simulink model "B2B_HVDC_MMC"  (R2023b)
settings: Solver=ode23t  StartTime=0.0  StopTime=3  FixedStep=Ts_Power  MaxStep=1e-3  MinStep=Ts_Power  RelTol=1e-3
values from neighbouring files (symbols this model uses):
  AC_lim = 1*[1.5 -1.5]    [B2B_HVDC_MMC_Calc.m]
  C_pm = 10.48e-3    (= 0.01048)    [B2B_HVDC_MMC_Calc.m]
  Carm = 1.0*C_pm/n    (= 0.0002096)    [B2B_HVDC_MMC_Calc.m]    (also in HVDC_MMC_param.m = 4.88333333333e-05)
  ccsc_lim = 1*[1.0 -1.0]    [B2B_HVDC_MMC_Calc.m]
  DC_lim = 1*[1.05 -1.05]    [B2B_HVDC_MMC_Calc.m]
  f = 50    [B2B_HVDC_MMC_Calc.m]
  Fn_filter = 1000    [B2B_HVDC_MMC_Calc.m]    (also in HVDC_MMC_param.m)
  Fnom = 50    [HVDC_MMC_param.m]
  HrmOrd = N    (= 2)    [B2B_HVDC_MMC_Calc.m]    (also in HVDC_MMC_param.m)
  I_nom = S_nom/(sqrt(3)*V_grid)    [B2B_HVDC_MMC_Calc.m]
  Ireg_lim_i = 1*[1.5, -1.5]    [B2B_HVDC_MMC_Calc.m]
  Ireg_lim_r = 2*[1.5, -1.5]    [B2B_HVDC_MMC_Calc.m]
  Ki_ACreg_i = 260    [B2B_HVDC_MMC_Calc.m]
  Ki_ccsc = 5    [B2B_HVDC_MMC_Calc.m]
  Ki_DCreg_r = 150    [B2B_HVDC_MMC_Calc.m]
  Ki_Ireg_i = 200    [B2B_HVDC_MMC_Calc.m]
  Ki_Ireg_r = 50    [B2B_HVDC_MMC_Calc.m]
  Kp_ACreg_i = 2    [B2B_HVDC_MMC_Calc.m]
  Kp_ccsc = 1    [B2B_HVDC_MMC_Calc.m]
  Kp_DCreg_r = 8    [B2B_HVDC_MMC_Calc.m]
  Kp_Ireg_i = 2    [B2B_HVDC_MMC_Calc.m]
  Kp_Ireg_r = 0.8    [B2B_HVDC_MMC_Calc.m]
  L1_si = L1_pu*Z_base66/w    [B2B_HVDC_MMC_Calc.m]
  L_arm = L_arm_pu*Z_base66/w    [B2B_HVDC_MMC_Calc.m]
  L_arm_pu = 0.15    [B2B_HVDC_MMC_Calc.m]
  N = 2    [B2B_HVDC_MMC_Calc.m]
  P_nom = 220e6    (= 220000000)    [B2B_HVDC_MMC_Calc.m]
  R1_si = R1_pu*Z_base66    [B2B_HVDC_MMC_Calc.m]
  R_arm = 0.03    [B2B_HVDC_MMC_Calc.m]
  R_arm_pu = R_arm/Z_base66    [B2B_HVDC_MMC_Calc.m]
  R_load = 0.6*40    (= 24)    [B2B_HVDC_MMC_Calc.m]
  R_startup = 17    [B2B_HVDC_MMC_Calc.m]    (also in HVDC_MMC_param.m = 400)
  T_fault = 1.4    [B2B_HVDC_MMC_Calc.m]
  Ts = Ts_Power    (= 5e-05)    [B2B_HVDC_MMC_Calc.m]    (also in HVDC_MMC_param.m)
  Ts_Control = Ts_Power    (= 5e-05)    [B2B_HVDC_MMC_Calc.m]    (also in HVDC_MMC_param.m)
  Ts_DQN = MultTs*Ts_Power    (= 5e-05)    [B2B_HVDC_MMC_Calc.m]    (also in HVDC_MMC_param.m)
  Ts_Power = 1*50e-6    (= 5e-05)    [B2B_HVDC_MMC_Calc.m]    (also in HVDC_MMC_param.m)
  V_ac_ref = 1.035    [B2B_HVDC_MMC_Calc.m]
  V_grid = 66e3    (= 66000)    [B2B_HVDC_MMC_Calc.m]
  Vdc_nom = 135e3    (= 135000)    [B2B_HVDC_MMC_Calc.m]
  Vnom_prim = 333e3    (= 333000)    [HVDC_MMC_param.m]
  Xdcpnz = [zeros(6,1), Xpnz]    [B2B_HVDC_MMC_Calc.m]
  Zeta_filter = 1    [B2B_HVDC_MMC_Calc.m]    (also in HVDC_MMC_param.m)
undefined symbols (not defined in the file or in its folder): DiscIntNeverNeededParam, Pcc, Xdcpnz_c
libraries: DQN_Lib x39, simulink x26, eeTransforms x21, spsCurrentMeasurementLib x16, spsHalfBridgeMMCLib x12, spsSeriesRLCBranchLib x12, B2B_HVDC_MMC_Lib x8, spsSecondOrderFilterLib x8, spsAlphaBetaZerotodq0Lib x6, spsabctoAlphaBetaZeroLib x6, spsThreePhaseVIMeasurementLib x4, spsabctodq0Lib x3
(part 4 of 5)

== system B2B_HVDC_MMC/Dq0 Control8/Subsystem/Circulating current suppression ==
  Id_dq2- : Inport
  Enable1 : EnablePort
  Constant1 : Constant  Value=0
  Constant2 : Constant  Value=0
  Constant4 : Constant  Value=0
  Demux : Demux  Outputs=2
  Discrete PID Controller : simulink/Continuous/PID Controller  Controller=PI  Form=Parallel  TimeDomain=Discrete-time  UseExternalTs=off  SampleTime=Ts_Power  IntegratorMethod=Forward Euler  ControllerParametersSource=internal  P=Kp_ccsc  I=Ki_ccsc  D=0  UseFilter=on  N=100  TunerSelectOption=Transfer Function Based (PID Tuner App)  InitialConditionSource=internal  InitialConditionForIntegrator=0  InitialConditionForFilter=0  DifferentiatorICPrevScaledInput=0  ExternalReset=none  TrackingMode=off  Kt=1  LimitOutput=off  UpperSaturationLimit=inf  LowerSaturationLimit=-inf  LinearizeAsGain=off  AntiWindupMode=none  Kb=1  POutMin=[]  POutMax=[]  IOutMin=[]  IOutMax=[]  DOutMin=[]  DOutMax=[]  NOutMin=[]  NOutMax=[]  SumOutMin=[]  SumOutMax=[]  SaturationOutMin=[]  SaturationOutMax=[]  PParamMin=[]  PParamMax=[]  IParamMin=[]  IParamMax=[]  DParamMin=[]  DParamMax=[]  NParamMin=[]  NParamMax=[]  KbParamMin=[]  KbParamMax=[]  KtParamMin=[]  KtParamMax=[]  KbOutMin=[]  KbOutMax=[]  KtOutMin=[]  KtOutMax=[]  IntegratorOutMin=[]  IntegratorOutMax=[]  FilterOutMin=[]  FilterOutMax=[]  SumI1OutMin=[]  SumI1OutMax=[]  SumI2OutMin=[]  SumI2OutMax=[]  SumI3OutMin=[]  SumI3OutMax=[]  SumI4OutMin=[]  SumI4OutMax=[]  SumDOutMin=[]  SumDOutMax=[]  DifferentiatorOutMin=[]  DifferentiatorOutMax=[]  FilterDiffOutCoefMin=[]  FilterDiffOutCoefMax=[]  ReciprocalOutMin=[]  ReciprocalOutMax=[]  SumDenOutMin=[]  SumDenOutMax=[]  SumNumOutMin=[]  SumNumOutMax=[]  DivideOutMin=[]  DivideOutMax=[]  UdiffTsProdOutMin=[]  UdiffTsProdOutMax=[]  NTsProdOutMin=[]  NTsProdOutMax=[]  UintegralTsProdOutMin=[]  UintegralTsProdOutMax=[]  UngainTsProdOutMin=[]  UngainTsProdOutMax=[]  IntegratorContinuousStateAttributes=''  IntegratorStateMustResolveToSignalObject=off  IntegratorRTWStateStorageClass=Auto  FilterContinuousStateAttributes=''  FilterStateMustResolveToSignalObject=off  FilterRTWStateStorageClass=Auto  ParallelPVariant=InternalParameters  IdealPVariant=Disabled  IVariant=InternalParameters  DVariant=Disabled  IntegratorVariant=Discrete  SatVariant=Disabled  AWVariant=Passthrough  PCopyVariant=Disabled  TRVariant=Disabled  FdbkBlocksVariant=Forward  IdealPFdbkVariant=Disabled  SatFdbkVariant=Disabled  DerivativeFilterVariant=Disabled  NVariant=Disabled  NCopyVariant=Disabled_SignalSpec  FilterICVariant=Disabled  IntegratorICVariant=InternalICs  ExternalResetVariant=Disabled  TRSumVariant=Passthrough  SumFdbkVariant=Disabled  SumVariant=Sum_PI  TsampFilterVariant=InternalTs  TsampNgainVariant=Passthrough  TsampIntegralVariant=Passthrough
  Discrete PID Controller1 : simulink/Continuous/PID Controller  Controller=PI  Form=Parallel  TimeDomain=Discrete-time  UseExternalTs=off  SampleTime=Ts_Power  IntegratorMethod=Forward Euler  ControllerParametersSource=internal  P=Kp_ccsc  I=Ki_ccsc  D=0  UseFilter=on  N=100  TunerSelectOption=Transfer Function Based (PID Tuner App)  InitialConditionSource=internal  InitialConditionForIntegrator=0  InitialConditionForFilter=0  DifferentiatorICPrevScaledInput=0  ExternalReset=none  TrackingMode=off  Kt=1  LimitOutput=off  UpperSaturationLimit=inf  LowerSaturationLimit=-inf  LinearizeAsGain=off  AntiWindupMode=none  Kb=1  POutMin=[]  POutMax=[]  IOutMin=[]  IOutMax=[]  DOutMin=[]  DOutMax=[]  NOutMin=[]  NOutMax=[]  SumOutMin=[]  SumOutMax=[]  SaturationOutMin=[]  SaturationOutMax=[]  PParamMin=[]  PParamMax=[]  IParamMin=[]  IParamMax=[]  DParamMin=[]  DParamMax=[]  NParamMin=[]  NParamMax=[]  KbParamMin=[]  KbParamMax=[]  KtParamMin=[]  KtParamMax=[]  KbOutMin=[]  KbOutMax=[]  KtOutMin=[]  KtOutMax=[]  IntegratorOutMin=[]  IntegratorOutMax=[]  FilterOutMin=[]  FilterOutMax=[]  SumI1OutMin=[]  SumI1OutMax=[]  SumI2OutMin=[]  SumI2OutMax=[]  SumI3OutMin=[]  SumI3OutMax=[]  SumI4OutMin=[]  SumI4OutMax=[]  SumDOutMin=[]  SumDOutMax=[]  DifferentiatorOutMin=[]  DifferentiatorOutMax=[]  FilterDiffOutCoefMin=[]  FilterDiffOutCoefMax=[]  ReciprocalOutMin=[]  ReciprocalOutMax=[]  SumDenOutMin=[]  SumDenOutMax=[]  SumNumOutMin=[]  SumNumOutMax=[]  DivideOutMin=[]  DivideOutMax=[]  UdiffTsProdOutMin=[]  UdiffTsProdOutMax=[]  NTsProdOutMin=[]  NTsProdOutMax=[]  UintegralTsProdOutMin=[]  UintegralTsProdOutMax=[]  UngainTsProdOutMin=[]  UngainTsProdOutMax=[]  IntegratorContinuousStateAttributes=''  IntegratorStateMustResolveToSignalObject=off  IntegratorRTWStateStorageClass=Auto  FilterContinuousStateAttributes=''  FilterStateMustResolveToSignalObject=off  FilterRTWStateStorageClass=Auto  ParallelPVariant=InternalParameters  IdealPVariant=Disabled  IVariant=InternalParameters  DVariant=Disabled  IntegratorVariant=Discrete  SatVariant=Disabled  AWVariant=Passthrough  PCopyVariant=Disabled  TRVariant=Disabled  FdbkBlocksVariant=Forward  IdealPFdbkVariant=Disabled  SatFdbkVariant=Disabled  DerivativeFilterVariant=Disabled  NVariant=Disabled  NCopyVariant=Disabled_SignalSpec  FilterICVariant=Disabled  IntegratorICVariant=InternalICs  ExternalResetVariant=Disabled  TRSumVariant=Passthrough  SumFdbkVariant=Disabled  SumVariant=Sum_PI  TsampFilterVariant=InternalTs  TsampNgainVariant=Passthrough  TsampIntegralVariant=Passthrough
  Gain : Gain  Gain=2*L_arm_pu
  Gain1 : Gain  Gain=2*L_arm_pu
  Mux1 : Mux  Inputs=3
  Sum1 : Sum  Inputs=-+|
  Sum78 : Sum  Inputs=|++
  Sum83 : Sum  Inputs=-+|
  Sum85 : Sum  Inputs=|+-
  m_dq2 : Outport  VectorParamsAs1DForOutWhenUnconnected=off
  wires:
  Constant2/1 -> Sum85/1
  Constant4/1 -> Mux1/3
  Sum1/1 -> Mux1/2
  Discrete PID Controller1/1 -> Sum1/2
  Discrete PID Controller/1 -> Sum78/1
  Id_dq2-/1 -> Demux/1
  Gain/1 -> Sum1/1
  Sum78/1 -> Mux1/1
  Sum85/1 -> Discrete PID Controller/1
  Sum83/1 -> Discrete PID Controller1/1
  Constant1/1 -> Sum83/2
  Demux/2 -> Sum83/1, Gain1/1
  Gain1/1 -> Sum78/2
  Demux/1 -> Sum85/2, Gain/1
  Mux1/1 -> m_dq2/1

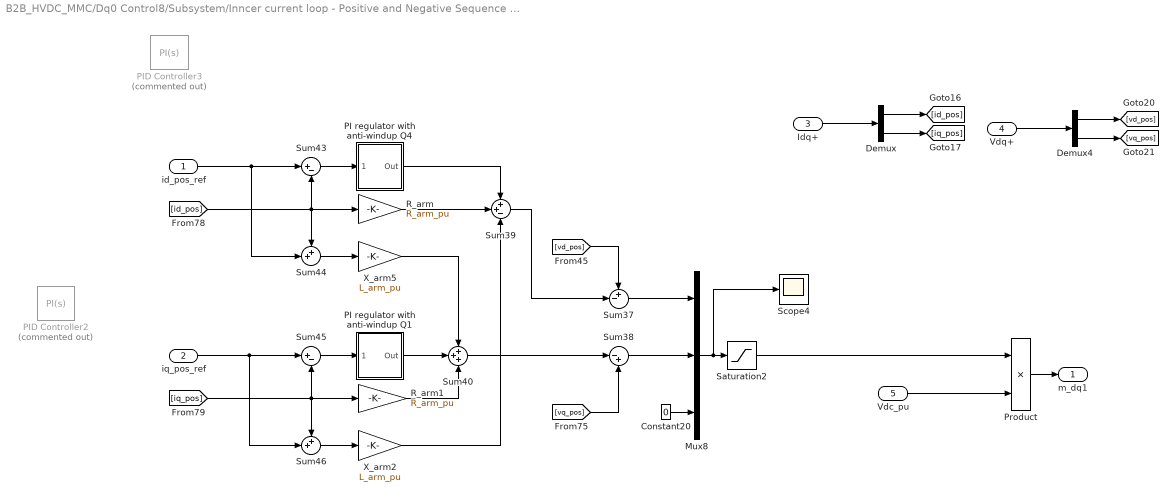
== system B2B_HVDC_MMC/Dq0 Control8/Subsystem/Inncer current loop - Positive and Negative Sequence Control ==
  id_pos_ref : Inport
  iq_pos_ref : Inport  Port=2
  Idq+ : Inport  Port=3
  Vdq+ : Inport  Port=4
  Vdc_pu : Inport  Port=5
  Constant20 : Constant  Value=0
  Demux : Demux  Outputs=2
  Demux4 : Demux  Outputs=2
  Mux8 : Mux  Inputs=3
  PI regulator with anti-windup Q1 : Subsystem  DialogController=POWERSYS.PowerSysDialog  mask(Discrete PI Controller){Kp=Kp_Ireg_i, Ki=Ki_Ireg_i, Par_Limits=[Ireg_lim_i(1) Ireg_lim_i(2)], Init=0, Ts=Ts_Control}
      mask prompts: Kp "Proportional gain (Kp):"; Ki "Integral gain (Ki):"; Par_Limits "Output limits: [ Upper   Lower ]"; Init "Output initial value:"; Ts "Sample time:"
      mask help: This block implements a discrete PI controller.
      mask init:
      | UpperLimit=Par_Limits(1);
      | LowerLimit=Par_Limits(2);
      | power_initmask();
      mask Help: This block is part of a subset of blocks in the Extras library that does not have documentation associated with it, other than the block mask description.
      mask Display: disp('PI');
  PI regulator with anti-windup Q4 : Subsystem  DialogController=POWERSYS.PowerSysDialog  mask(Discrete PI Controller){Kp=Kp_Ireg_i, Ki=Ki_Ireg_i, Par_Limits=[Ireg_lim_i(1) Ireg_lim_i(2)], Init=0, Ts=Ts_Control}
      mask prompts: Kp "Proportional gain (Kp):"; Ki "Integral gain (Ki):"; Par_Limits "Output limits: [ Upper   Lower ]"; Init "Output initial value:"; Ts "Sample time:"
      mask help: This block implements a discrete PI controller.
      mask init:
      | UpperLimit=Par_Limits(1);
      | LowerLimit=Par_Limits(2);
      | power_initmask();
      mask Help: This block is part of a subset of blocks in the Extras library that does not have documentation associated with it, other than the block mask description.
      mask Display: disp('PI');
  PID Controller2 : simulink/Continuous/PID Controller  Commented=on  Controller=PI  Form=Parallel  TimeDomain=Continuous-time  UseExternalTs=off  SampleTime=-1  IntegratorMethod=Forward Euler  ControllerParametersSource=internal  P=Kp_Ireg_i  I=Ki_Ireg_i  D=0  UseFilter=on  N=100  TunerSelectOption=Transfer Function Based (PID Tuner App)  InitialConditionSource=internal  InitialConditionForIntegrator=0  InitialConditionForFilter=0  DifferentiatorICPrevScaledInput=0  ExternalReset=none  TrackingMode=off  Kt=1  LimitOutput=off  UpperSaturationLimit=inf  LowerSaturationLimit=-inf  LinearizeAsGain=on  AntiWindupMode=none  Kb=1  POutMin=[]  POutMax=[]  IOutMin=[]  IOutMax=[]  DOutMin=[]  DOutMax=[]  NOutMin=[]  NOutMax=[]  SumOutMin=[]  SumOutMax=[]  SaturationOutMin=[]  SaturationOutMax=[]  PParamMin=[]  PParamMax=[]  IParamMin=[]  IParamMax=[]  DParamMin=[]  DParamMax=[]  NParamMin=[]  NParamMax=[]  KbParamMin=[]  KbParamMax=[]  KtParamMin=[]  KtParamMax=[]  KbOutMin=[]  KbOutMax=[]  KtOutMin=[]  KtOutMax=[]  IntegratorOutMin=[]  IntegratorOutMax=[]  FilterOutMin=[]  FilterOutMax=[]  SumI1OutMin=[]  SumI1OutMax=[]  SumI2OutMin=[]  SumI2OutMax=[]  SumI3OutMin=[]  SumI3OutMax=[]  SumI4OutMin=[]  SumI4OutMax=[]  SumDOutMin=[]  SumDOutMax=[]  DifferentiatorOutMin=[]  DifferentiatorOutMax=[]  FilterDiffOutCoefMin=[]  FilterDiffOutCoefMax=[]  ReciprocalOutMin=[]  ReciprocalOutMax=[]  SumDenOutMin=[]  SumDenOutMax=[]  SumNumOutMin=[]  SumNumOutMax=[]  DivideOutMin=[]  DivideOutMax=[]  UdiffTsProdOutMin=[]  UdiffTsProdOutMax=[]  NTsProdOutMin=[]  NTsProdOutMax=[]  UintegralTsProdOutMin=[]  UintegralTsProdOutMax=[]  UngainTsProdOutMin=[]  UngainTsProdOutMax=[]  IntegratorContinuousStateAttributes=''  IntegratorStateMustResolveToSignalObject=off  IntegratorRTWStateStorageClass=Auto  FilterContinuousStateAttributes=''  FilterStateMustResolveToSignalObject=off  FilterRTWStateStorageClass=Auto  ParallelPVariant=InternalParameters  IdealPVariant=Disabled  IVariant=InternalParameters  DVariant=Disabled  IntegratorVariant=Continuous  SatVariant=Disabled  AWVariant=Passthrough  PCopyVariant=Disabled  TRVariant=Disabled  FdbkBlocksVariant=Forward  IdealPFdbkVariant=Disabled  SatFdbkVariant=Disabled  DerivativeFilterVariant=Disabled  NVariant=Disabled  NCopyVariant=Disabled_SignalSpec  FilterICVariant=Disabled  IntegratorICVariant=InternalICs  ExternalResetVariant=Disabled  TRSumVariant=Passthrough  SumFdbkVariant=Disabled  SumVariant=Sum_PI  TsampFilterVariant=InternalTs  TsampNgainVariant=Passthrough  TsampIntegralVariant=Passthrough
  PID Controller3 : simulink/Continuous/PID Controller  Commented=on  Controller=PI  Form=Parallel  TimeDomain=Continuous-time  UseExternalTs=off  SampleTime=-1  IntegratorMethod=Forward Euler  ControllerParametersSource=internal  P=Kp_Ireg_i  I=Ki_Ireg_i  D=0  UseFilter=on  N=100  TunerSelectOption=Transfer Function Based (PID Tuner App)  InitialConditionSource=internal  InitialConditionForIntegrator=0  InitialConditionForFilter=0  DifferentiatorICPrevScaledInput=0  ExternalReset=none  TrackingMode=off  Kt=1  LimitOutput=off  UpperSaturationLimit=inf  LowerSaturationLimit=-inf  LinearizeAsGain=on  AntiWindupMode=none  Kb=1  POutMin=[]  POutMax=[]  IOutMin=[]  IOutMax=[]  DOutMin=[]  DOutMax=[]  NOutMin=[]  NOutMax=[]  SumOutMin=[]  SumOutMax=[]  SaturationOutMin=[]  SaturationOutMax=[]  PParamMin=[]  PParamMax=[]  IParamMin=[]  IParamMax=[]  DParamMin=[]  DParamMax=[]  NParamMin=[]  NParamMax=[]  KbParamMin=[]  KbParamMax=[]  KtParamMin=[]  KtParamMax=[]  KbOutMin=[]  KbOutMax=[]  KtOutMin=[]  KtOutMax=[]  IntegratorOutMin=[]  IntegratorOutMax=[]  FilterOutMin=[]  FilterOutMax=[]  SumI1OutMin=[]  SumI1OutMax=[]  SumI2OutMin=[]  SumI2OutMax=[]  SumI3OutMin=[]  SumI3OutMax=[]  SumI4OutMin=[]  SumI4OutMax=[]  SumDOutMin=[]  SumDOutMax=[]  DifferentiatorOutMin=[]  DifferentiatorOutMax=[]  FilterDiffOutCoefMin=[]  FilterDiffOutCoefMax=[]  ReciprocalOutMin=[]  ReciprocalOutMax=[]  SumDenOutMin=[]  SumDenOutMax=[]  SumNumOutMin=[]  SumNumOutMax=[]  DivideOutMin=[]  DivideOutMax=[]  UdiffTsProdOutMin=[]  UdiffTsProdOutMax=[]  NTsProdOutMin=[]  NTsProdOutMax=[]  UintegralTsProdOutMin=[]  UintegralTsProdOutMax=[]  UngainTsProdOutMin=[]  UngainTsProdOutMax=[]  IntegratorContinuousStateAttributes=''  IntegratorStateMustResolveToSignalObject=off  IntegratorRTWStateStorageClass=Auto  FilterContinuousStateAttributes=''  FilterStateMustResolveToSignalObject=off  FilterRTWStateStorageClass=Auto  ParallelPVariant=InternalParameters  IdealPVariant=Disabled  IVariant=InternalParameters  DVariant=Disabled  IntegratorVariant=Continuous  SatVariant=Disabled  AWVariant=Passthrough  PCopyVariant=Disabled  TRVariant=Disabled  FdbkBlocksVariant=Forward  IdealPFdbkVariant=Disabled  SatFdbkVariant=Disabled  DerivativeFilterVariant=Disabled  NVariant=Disabled  NCopyVariant=Disabled_SignalSpec  FilterICVariant=Disabled  IntegratorICVariant=InternalICs  ExternalResetVariant=Disabled  TRSumVariant=Passthrough  SumFdbkVariant=Disabled  SumVariant=Sum_PI  TsampFilterVariant=InternalTs  TsampNgainVariant=Passthrough  TsampIntegralVariant=Passthrough
  Product : Product
  R_arm : Gain  Gain=R_arm_pu
  R_arm1 : Gain  Gain=R_arm_pu
  Saturation2 : Saturate  UpperLimit=Ireg_lim_i(1)  LowerLimit=Ireg_lim_i(2)
  Scope4 : Scope
  Sum37 : Sum  Inputs=+-|
  Sum38 : Sum  Inputs=|-+
  Sum39 : Sum  Inputs=++-
  Sum40 : Sum  Inputs=+++
  Sum43 : Sum  Inputs=|+-
  Sum44 : Sum  Inputs=++|
  Sum45 : Sum  Inputs=|+-
  Sum46 : Sum  Inputs=++|
  X_arm2 : Gain  Gain=L_arm_pu
  X_arm5 : Gain  Gain=L_arm_pu
  m_dq1 : Outport  VectorParamsAs1DForOutWhenUnconnected=off
  wires:
  Mux8/1 -> Scope4/1, Saturation2/1
  Vdq+/1 -> Demux4/1
  Idq+/1 -> Demux/1
  [id_pos] -> Sum44/1, Sum43/2, R_arm/1
  Demux4/2 -> [vq_pos]
  Demux4/1 -> [vd_pos]
  Demux/1 -> [id_pos]
  Demux/2 -> [iq_pos]
  Sum45/1 -> PI regulator with anti-windup Q1/1(Error)
  Sum37/1 -> Mux8/1
  iq_pos_ref/1 -> Sum45/1, Sum46/2
  Sum40/1 -> Sum38/1
  X_arm2/1 -> Sum39/3
  R_arm1/1 -> Sum40/3
  R_arm/1 -> Sum39/2
  Sum44/1 -> X_arm5/1
  Sum43/1 -> PI regulator with anti-windup Q4/1(Error)
  Sum46/1 -> X_arm2/1
  Sum38/1 -> Mux8/2
  [vd_pos] -> Sum37/1
  [vq_pos] -> Sum38/2
  X_arm5/1 -> Sum40/1
  Sum39/1 -> Sum37/2
  id_pos_ref/1 -> Sum43/1, Sum44/2
  PI regulator with anti-windup Q1/1(Out) -> Sum40/2
  Constant20/1 -> Mux8/3
  [iq_pos] -> Sum45/2, Sum46/1, R_arm1/1
  PI regulator with anti-windup Q4/1(Out) -> Sum39/1
  Vdc_pu/1 -> Product/2
  Saturation2/1 -> Product/1
  Product/1 -> m_dq1/1

== system B2B_HVDC_MMC/Dq0 Control8/Subsystem/Outer loop - AC RMS controller1 ==
  Vac_ref : Inport
  vdq+ : Inport  Port=2
  Enable : Inport  Port=3
  PI regulator with anti-windup Q1 : Subsystem  DialogController=POWERSYS.PowerSysDialog  mask(Discrete PI Controller){Kp=Kp_ACreg_i, Ki=Ki_ACreg_i, Par_Limits=[AC_lim(1) AC_lim(2)], Init=0, Ts=Ts_Control}
      mask prompts: Kp "Proportional gain (Kp):"; Ki "Integral gain (Ki):"; Par_Limits "Output limits: [ Upper   Lower ]"; Init "Output initial value:"; Ts "Sample time:"
      mask help: This block implements a discrete PI controller.
      mask init:
      | UpperLimit=Par_Limits(1);
      | LowerLimit=Par_Limits(2);
      | power_initmask();
      mask Help: This block is part of a subset of blocks in the Extras library that does not have documentation associated with it, other than the block mask description.
      mask Display: disp('PI');
  Selector : Selector  InputPortWidth=2  IndexOptions=Index vector (dialog)  Indices=[1]  OutputSizes=1
  Sum1 : Sum  Inputs=|+-
  Switch1 : Switch  Criteria=u2 > Threshold  Threshold=0.5  OutDataTypeStr=double  SaturateOnIntegerOverflow=off  InputSameDT=off
  Id_ref : Outport  VectorParamsAs1DForOutWhenUnconnected=off
  wires:
  vdq+/1 -> Selector/1
  Sum1/1 -> PI regulator with anti-windup Q1/1(Error)
  Enable/1 -> Switch1/2
  Switch1/1 -> Sum1/1
  Vac_ref/1 -> Switch1/1
  PI regulator with anti-windup Q1/1(Out) -> [Idp_ref], Id_ref/1
  Selector/1 -> Switch1/3, Sum1/2

== system B2B_HVDC_MMC/Dq0 Control8/Subsystem/Reactive power Set-point ==
  T_Qreg_on : Inport
  Q_ref : Inport  Port=2
  Vdq+ : Inport  Port=3
  Enable : EnablePort
  Constant : Constant  Value=0
  Constant1 : Constant
  Constant2 : Constant  Value=0.75
  Divide : Product  Inputs=*/
  Gain3 : Gain  Gain=-1
  Rate Transition9 : RateTransition  Commented=on  OutPortSampleTime=Ts_Control
  Scope : Scope  NumInputPorts=4
  Selector : Selector  InputPortWidth=2  IndexOptions=Index vector (dialog)  Indices=[1]  OutputSizes=1
  Selector1 : Selector  InputPortWidth=2  IndexOptions=Index vector (dialog)  Indices=[2]  OutputSizes=1
  Switch : Switch  Criteria=u2 > Threshold  SaturateOnIntegerOverflow=off  InputSameDT=off
  Switch1 : Switch  Criteria=u2 > Threshold  SaturateOnIntegerOverflow=off  InputSameDT=off
  Switch2 : Switch  Criteria=u2 > Threshold  Threshold=0.65  SaturateOnIntegerOverflow=off  InputSameDT=off
  Unit Delay6 : UnitDelay  Commented=on  SampleTime=Ts_Power  HasFrameUpgradeWarning=on
  Iq_ref : Outport  VectorParamsAs1DForOutWhenUnconnected=off
  wires:
  Switch/1 -> Divide/1
  Vdq+/1 -> Selector/1
  Switch1/1 -> Divide/2, Scope/2
  Constant/1 -> Switch/3
  Divide/1 -> Gain3/1
  Selector1/1 -> Switch/1
  Q_ref/1 -> Selector1/1
  Constant1/1 -> Switch1/3
  T_Qreg_on/1 -> Switch1/2, Switch/2
  Constant2/1 -> Switch2/3
  Selector/1 -> Switch2/2, Switch2/1, Scope/3
  Unit Delay6/1 -> Rate Transition9/1
  Gain3/1 -> Scope/1, [Iqp_ref], Iq_ref/1
  Switch2/1 -> Switch1/1

== system B2B_HVDC_MMC/Dq0 Control11/Subsystem1/DC voltage control - Outer loop/PI regulator with anti-windup Q ==
  note: Anti-windup mechanism: Method of conditionnal integration
      |
      | The integration is suspended if saturation occurs and the
      | control error is of the same sign as the control signal.
      |
      | [1] L.Rundqwist, "Anti-Reset Windup for PID Controllers," Ph.D. Thesis TRFT-1033,
      | Departement of Automatic Control, Lund Institute of Technology, Lund, Sweeden, 1991.
  note: Modified by Tony - Adding controllable saturation operation for fault handling.
  Error : Inport  SampleTime=Ts
  Limit : Inport  Port=2
  Compare To Zero : simulink/Logic and Bit Operations/Compare To Zero  relop=>  OutDataTypeStr=uint8  ZeroCross=off
  Compare To Zero1 : simulink/Logic and Bit Operations/Compare To Zero  relop=<  OutDataTypeStr=uint8  ZeroCross=off
  Constant : Constant  Value=0
  Constant2 : Constant  Value=UpperLimit
  Constant3 : Constant  Value=LowerLimit
  Demux : Demux  Outputs=2
  Discrete-Time Integrator1 : DiscreteIntegrator  IntegratorMethod=Integration: Trapezoidal  InitialCondition=Init  SampleTime=Ts  LimitOutput=on  UpperSaturationLimit=UpperLimit  LowerSaturationLimit=LowerLimit  ShowStatePort=on  ICPrevOutput=DiscIntNeverNeededParam  ICPrevScaledInput=DiscIntNeverNeededParam
  Kp4 : Gain  Gain=Kp  SaturateOnIntegerOverflow=on  SampleTime=Ts  OutDataTypeStr=Inherit: Same as input  ParamDataTypeStr=Inherit: Same as input
  Kp5 : Gain  Gain=Ki  SaturateOnIntegerOverflow=on  SampleTime=Ts  OutDataTypeStr=Inherit: Same as input  ParamDataTypeStr=Inherit: Same as input
  Logical Operator : Logic  AllPortsSameDT=off  OutDataTypeStr=boolean
  Logical Operator1 : Logic  AllPortsSameDT=off  OutDataTypeStr=boolean
  Logical Operator2 : Logic  Operator=OR  AllPortsSameDT=off  OutDataTypeStr=boolean
  Relational Operator : RelationalOperator  OutDataTypeStr=boolean  InputSameDT=off
  Relational Operator1 : RelationalOperator  Operator=<=  OutDataTypeStr=boolean  InputSameDT=off
  Saturation Dynamic1 : simulink/Discontinuities/Saturation Dynamic  OutMin=[]  OutMax=[]  OutDataTypeStr=Inherit: Same as second input  OutDataType=fixdt(1, 16)  OutScaling=2^-10  DoSatur=off
  Sum1 : Sum  InputSameDT=on  SaturateOnIntegerOverflow=on  SampleTime=Ts  OutDataTypeStr=Inherit: Same as first input
  Sum6 : Sum  InputSameDT=on  SaturateOnIntegerOverflow=on  SampleTime=Ts  OutDataTypeStr=Inherit: Same as first input
  Switch : Switch  Criteria=u2 > Threshold  SaturateOnIntegerOverflow=off  InputSameDT=off
  Zero-Order Hold : ZeroOrderHold  SampleTime=Ts
  Out : Outport  SampleTime=Ts  InitialOutput=0  VectorParamsAs1DForOutWhenUnconnected=off
  wires:
  Constant3/1 -> Relational Operator1/2
  Constant2/1 -> Relational Operator/2
  Saturation Dynamic1/1 -> Out/1
  Sum6/1 -> Saturation Dynamic1/2
  Discrete-Time Integrator1/State -> Sum1/1
  Discrete-Time Integrator1/1 -> Sum6/2
  Constant/1 -> Switch/1
  Zero-Order Hold/1 -> Sum1/2, Sum6/1
  Sum1/1 -> Relational Operator1/1, Relational Operator/1
  Logical Operator2/1 -> Switch/2
  Relational Operator/1 -> Logical Operator/1  "UpperLimit_is_Reached"
  Relational Operator1/1 -> Logical Operator1/1  "LowerLimit_Is_Reached"
  Compare To Zero/1 -> Logical Operator/2  "Error_is_positive"
  Logical Operator/1 -> Logical Operator2/1
  Logical Operator1/1 -> Logical Operator2/2
  Compare To Zero1/1 -> Logical Operator1/2  "Error_is_negative"
  Error/1 -> Compare To Zero1/1, Compare To Zero/1, Kp4/1, Kp5/1
  Kp4/1 -> Zero-Order Hold/1
  Switch/1 -> Discrete-Time Integrator1/1
  Kp5/1 -> Switch/3
  Limit/1 -> Demux/1
  Demux/1 -> Saturation Dynamic1/1
  Demux/2 -> Saturation Dynamic1/3

== system B2B_HVDC_MMC/Dq0 Control11/Subsystem1/Inncer current loop - Positive and Negative Sequence Control/PI regulator with anti-windup Q1 ==
  note: Anti-windup mechanism: Method of conditionnal integration
      |
      | The integration is suspended if saturation occurs and the
      | control error is of the same sign as the control signal.
      |
      | [1] L.Rundqwist, "Anti-Reset Windup for PID Controllers," Ph.D. Thesis TRFT-1033,
      | Departement of Automatic Control, Lund Institute of Technology, Lund, Sweeden, 1991.
  Error : Inport  SampleTime=Ts
  Compare To Zero : simulink/Logic and Bit Operations/Compare To Zero  relop=>  OutDataTypeStr=uint8  ZeroCross=off
  Compare To Zero1 : simulink/Logic and Bit Operations/Compare To Zero  relop=<  OutDataTypeStr=uint8  ZeroCross=off
  Constant : Constant  Value=0
  Constant1 : Constant  Value=UpperLimit
  Constant3 : Constant  Value=LowerLimit
  Discrete-Time Integrator : DiscreteIntegrator  IntegratorMethod=Integration: Trapezoidal  InitialCondition=Init  SampleTime=Ts  LimitOutput=on  UpperSaturationLimit=UpperLimit  LowerSaturationLimit=LowerLimit  ShowStatePort=on  ICPrevOutput=DiscIntNeverNeededParam  ICPrevScaledInput=DiscIntNeverNeededParam
  Kp4 : Gain  Gain=Kp  SaturateOnIntegerOverflow=on  SampleTime=Ts  OutDataTypeStr=Inherit: Same as input  ParamDataTypeStr=Inherit: Same as input
  Kp5 : Gain  Gain=Ki  SaturateOnIntegerOverflow=on  SampleTime=Ts  OutDataTypeStr=Inherit: Same as input  ParamDataTypeStr=Inherit: Same as input
  Logical Operator : Logic  AllPortsSameDT=off  OutDataTypeStr=boolean
  Logical Operator1 : Logic  AllPortsSameDT=off  OutDataTypeStr=boolean
  Logical Operator2 : Logic  Operator=OR  AllPortsSameDT=off  OutDataTypeStr=boolean
  Relational Operator : RelationalOperator  OutDataTypeStr=boolean  InputSameDT=off
  Relational Operator1 : RelationalOperator  Operator=<=  OutDataTypeStr=boolean  InputSameDT=off
  Saturation2 : Saturate  UpperLimit=UpperLimit  LowerLimit=LowerLimit  SampleTime=Ts
  Sum1 : Sum  InputSameDT=on  SaturateOnIntegerOverflow=on  SampleTime=Ts  OutDataTypeStr=Inherit: Same as first input
  Sum6 : Sum  InputSameDT=on  SaturateOnIntegerOverflow=on  SampleTime=Ts  OutDataTypeStr=Inherit: Same as first input
  Switch : Switch  Criteria=u2 > Threshold  SaturateOnIntegerOverflow=off  InputSameDT=off
  Zero-Order Hold : ZeroOrderHold  SampleTime=Ts
  Out : Outport  SampleTime=Ts  InitialOutput=0  VectorParamsAs1DForOutWhenUnconnected=off
  wires:
  Kp5/1 -> Switch/3
  Switch/1 -> Discrete-Time Integrator/1
  Saturation2/1 -> Out/1
  Discrete-Time Integrator/1 -> Sum6/2
  Kp4/1 -> Zero-Order Hold/1
  Sum6/1 -> Saturation2/1
  Error/1 -> Kp5/1, Kp4/1, Compare To Zero/1, Compare To Zero1/1
  Compare To Zero1/1 -> Logical Operator1/2  "Error_is_negative"
  Logical Operator1/1 -> Logical Operator2/2
  Logical Operator/1 -> Logical Operator2/1
  Compare To Zero/1 -> Logical Operator/2  "Error_is_positive"
  Constant3/1 -> Relational Operator1/2
  Constant1/1 -> Relational Operator/2
  Relational Operator1/1 -> Logical Operator1/1  "LowerLimit_Is_Reached"
  Relational Operator/1 -> Logical Operator/1  "UpperLimit_is_Reached"
  Logical Operator2/1 -> Switch/2
  Sum1/1 -> Relational Operator/1, Relational Operator1/1
  Discrete-Time Integrator/State -> Sum1/1
  Zero-Order Hold/1 -> Sum6/1, Sum1/2
  Constant/1 -> Switch/1

== system B2B_HVDC_MMC/Dq0 Control11/Subsystem1/Inncer current loop - Positive and Negative Sequence Control/PI regulator with anti-windup Q4 ==
  note: Anti-windup mechanism: Method of conditionnal integration
      |
      | The integration is suspended if saturation occurs and the
      | control error is of the same sign as the control signal.
      |
      | [1] L.Rundqwist, "Anti-Reset Windup for PID Controllers," Ph.D. Thesis TRFT-1033,
      | Departement of Automatic Control, Lund Institute of Technology, Lund, Sweeden, 1991.
  Error : Inport  SampleTime=Ts
  Compare To Zero : simulink/Logic and Bit Operations/Compare To Zero  relop=>  OutDataTypeStr=uint8  ZeroCross=off
  Compare To Zero1 : simulink/Logic and Bit Operations/Compare To Zero  relop=<  OutDataTypeStr=uint8  ZeroCross=off
  Constant : Constant  Value=0
  Constant1 : Constant  Value=UpperLimit
  Constant3 : Constant  Value=LowerLimit
  Discrete-Time Integrator : DiscreteIntegrator  IntegratorMethod=Integration: Trapezoidal  InitialCondition=Init  SampleTime=Ts  LimitOutput=on  UpperSaturationLimit=UpperLimit  LowerSaturationLimit=LowerLimit  ShowStatePort=on  ICPrevOutput=DiscIntNeverNeededParam  ICPrevScaledInput=DiscIntNeverNeededParam
  Kp4 : Gain  Gain=Kp  SaturateOnIntegerOverflow=on  SampleTime=Ts  OutDataTypeStr=Inherit: Same as input  ParamDataTypeStr=Inherit: Same as input
  Kp5 : Gain  Gain=Ki  SaturateOnIntegerOverflow=on  SampleTime=Ts  OutDataTypeStr=Inherit: Same as input  ParamDataTypeStr=Inherit: Same as input
  Logical Operator : Logic  AllPortsSameDT=off  OutDataTypeStr=boolean
  Logical Operator1 : Logic  AllPortsSameDT=off  OutDataTypeStr=boolean
  Logical Operator2 : Logic  Operator=OR  AllPortsSameDT=off  OutDataTypeStr=boolean
  Relational Operator : RelationalOperator  OutDataTypeStr=boolean  InputSameDT=off
  Relational Operator1 : RelationalOperator  Operator=<=  OutDataTypeStr=boolean  InputSameDT=off
  Saturation2 : Saturate  UpperLimit=UpperLimit  LowerLimit=LowerLimit  SampleTime=Ts
  Sum1 : Sum  InputSameDT=on  SaturateOnIntegerOverflow=on  SampleTime=Ts  OutDataTypeStr=Inherit: Same as first input
  Sum6 : Sum  InputSameDT=on  SaturateOnIntegerOverflow=on  SampleTime=Ts  OutDataTypeStr=Inherit: Same as first input
  Switch : Switch  Criteria=u2 > Threshold  SaturateOnIntegerOverflow=off  InputSameDT=off
  Zero-Order Hold : ZeroOrderHold  SampleTime=Ts
  Out : Outport  SampleTime=Ts  InitialOutput=0  VectorParamsAs1DForOutWhenUnconnected=off
  wires:
  Kp5/1 -> Switch/3
  Switch/1 -> Discrete-Time Integrator/1
  Saturation2/1 -> Out/1
  Discrete-Time Integrator/1 -> Sum6/2
  Kp4/1 -> Zero-Order Hold/1
  Sum6/1 -> Saturation2/1
  Error/1 -> Kp5/1, Kp4/1, Compare To Zero/1, Compare To Zero1/1
  Compare To Zero1/1 -> Logical Operator1/2  "Error_is_negative"
  Logical Operator1/1 -> Logical Operator2/2
  Logical Operator/1 -> Logical Operator2/1
  Compare To Zero/1 -> Logical Operator/2  "Error_is_positive"
  Constant3/1 -> Relational Operator1/2
  Constant1/1 -> Relational Operator/2
  Relational Operator1/1 -> Logical Operator1/1  "LowerLimit_Is_Reached"
  Relational Operator/1 -> Logical Operator/1  "UpperLimit_is_Reached"
  Logical Operator2/1 -> Switch/2
  Sum1/1 -> Relational Operator/1, Relational Operator1/1
  Discrete-Time Integrator/State -> Sum1/1
  Zero-Order Hold/1 -> Sum6/1, Sum1/2
  Constant/1 -> Switch/1

== system B2B_HVDC_MMC/Dq0 Control8/Subsystem/Inncer current loop - Positive and Negative Sequence Control/PI regulator with anti-windup Q1 ==
  note: Anti-windup mechanism: Method of conditionnal integration
      |
      | The integration is suspended if saturation occurs and the
      | control error is of the same sign as the control signal.
      |
      | [1] L.Rundqwist, "Anti-Reset Windup for PID Controllers," Ph.D. Thesis TRFT-1033,
      | Departement of Automatic Control, Lund Institute of Technology, Lund, Sweeden, 1991.
  Error : Inport  SampleTime=Ts
  Compare To Zero : simulink/Logic and Bit Operations/Compare To Zero  relop=>  OutDataTypeStr=uint8  ZeroCross=off
  Compare To Zero1 : simulink/Logic and Bit Operations/Compare To Zero  relop=<  OutDataTypeStr=uint8  ZeroCross=off
  Constant : Constant  Value=0
  Constant1 : Constant  Value=UpperLimit
  Constant3 : Constant  Value=LowerLimit
  Discrete-Time Integrator : DiscreteIntegrator  IntegratorMethod=Integration: Trapezoidal  InitialCondition=Init  SampleTime=Ts  LimitOutput=on  UpperSaturationLimit=UpperLimit  LowerSaturationLimit=LowerLimit  ShowStatePort=on  ICPrevOutput=DiscIntNeverNeededParam  ICPrevScaledInput=DiscIntNeverNeededParam
  Kp4 : Gain  Gain=Kp  SaturateOnIntegerOverflow=on  SampleTime=Ts  OutDataTypeStr=Inherit: Same as input  ParamDataTypeStr=Inherit: Same as input
  Kp5 : Gain  Gain=Ki  SaturateOnIntegerOverflow=on  SampleTime=Ts  OutDataTypeStr=Inherit: Same as input  ParamDataTypeStr=Inherit: Same as input
  Logical Operator : Logic  AllPortsSameDT=off  OutDataTypeStr=boolean
  Logical Operator1 : Logic  AllPortsSameDT=off  OutDataTypeStr=boolean
  Logical Operator2 : Logic  Operator=OR  AllPortsSameDT=off  OutDataTypeStr=boolean
  Relational Operator : RelationalOperator  OutDataTypeStr=boolean  InputSameDT=off
  Relational Operator1 : RelationalOperator  Operator=<=  OutDataTypeStr=boolean  InputSameDT=off
  Saturation2 : Saturate  UpperLimit=UpperLimit  LowerLimit=LowerLimit  SampleTime=Ts
  Sum1 : Sum  InputSameDT=on  SaturateOnIntegerOverflow=on  SampleTime=Ts  OutDataTypeStr=Inherit: Same as first input
  Sum6 : Sum  InputSameDT=on  SaturateOnIntegerOverflow=on  SampleTime=Ts  OutDataTypeStr=Inherit: Same as first input
  Switch : Switch  Criteria=u2 > Threshold  SaturateOnIntegerOverflow=off  InputSameDT=off
  Zero-Order Hold : ZeroOrderHold  SampleTime=Ts
  Out : Outport  SampleTime=Ts  InitialOutput=0  VectorParamsAs1DForOutWhenUnconnected=off
  wires:
  Kp5/1 -> Switch/3
  Switch/1 -> Discrete-Time Integrator/1
  Saturation2/1 -> Out/1
  Discrete-Time Integrator/1 -> Sum6/2
  Kp4/1 -> Zero-Order Hold/1
  Sum6/1 -> Saturation2/1
  Error/1 -> Kp5/1, Kp4/1, Compare To Zero/1, Compare To Zero1/1
  Compare To Zero1/1 -> Logical Operator1/2  "Error_is_negative"
  Logical Operator1/1 -> Logical Operator2/2
  Logical Operator/1 -> Logical Operator2/1
  Compare To Zero/1 -> Logical Operator/2  "Error_is_positive"
  Constant3/1 -> Relational Operator1/2
  Constant1/1 -> Relational Operator/2
  Relational Operator1/1 -> Logical Operator1/1  "LowerLimit_Is_Reached"
  Relational Operator/1 -> Logical Operator/1  "UpperLimit_is_Reached"
  Logical Operator2/1 -> Switch/2
  Sum1/1 -> Relational Operator/1, Relational Operator1/1
  Discrete-Time Integrator/State -> Sum1/1
  Zero-Order Hold/1 -> Sum6/1, Sum1/2
  Constant/1 -> Switch/1

== system B2B_HVDC_MMC/Dq0 Control8/Subsystem/Inncer current loop - Positive and Negative Sequence Control/PI regulator with anti-windup Q4 ==
  note: Anti-windup mechanism: Method of conditionnal integration
      |
      | The integration is suspended if saturation occurs and the
      | control error is of the same sign as the control signal.
      |
      | [1] L.Rundqwist, "Anti-Reset Windup for PID Controllers," Ph.D. Thesis TRFT-1033,
      | Departement of Automatic Control, Lund Institute of Technology, Lund, Sweeden, 1991.
  Error : Inport  SampleTime=Ts
  Compare To Zero : simulink/Logic and Bit Operations/Compare To Zero  relop=>  OutDataTypeStr=uint8  ZeroCross=off
  Compare To Zero1 : simulink/Logic and Bit Operations/Compare To Zero  relop=<  OutDataTypeStr=uint8  ZeroCross=off
  Constant : Constant  Value=0
  Constant1 : Constant  Value=UpperLimit
  Constant3 : Constant  Value=LowerLimit
  Discrete-Time Integrator : DiscreteIntegrator  IntegratorMethod=Integration: Trapezoidal  InitialCondition=Init  SampleTime=Ts  LimitOutput=on  UpperSaturationLimit=UpperLimit  LowerSaturationLimit=LowerLimit  ShowStatePort=on  ICPrevOutput=DiscIntNeverNeededParam  ICPrevScaledInput=DiscIntNeverNeededParam
  Kp4 : Gain  Gain=Kp  SaturateOnIntegerOverflow=on  SampleTime=Ts  OutDataTypeStr=Inherit: Same as input  ParamDataTypeStr=Inherit: Same as input
  Kp5 : Gain  Gain=Ki  SaturateOnIntegerOverflow=on  SampleTime=Ts  OutDataTypeStr=Inherit: Same as input  ParamDataTypeStr=Inherit: Same as input
  Logical Operator : Logic  AllPortsSameDT=off  OutDataTypeStr=boolean
  Logical Operator1 : Logic  AllPortsSameDT=off  OutDataTypeStr=boolean
  Logical Operator2 : Logic  Operator=OR  AllPortsSameDT=off  OutDataTypeStr=boolean
  Relational Operator : RelationalOperator  OutDataTypeStr=boolean  InputSameDT=off
  Relational Operator1 : RelationalOperator  Operator=<=  OutDataTypeStr=boolean  InputSameDT=off
  Saturation2 : Saturate  UpperLimit=UpperLimit  LowerLimit=LowerLimit  SampleTime=Ts
  Sum1 : Sum  InputSameDT=on  SaturateOnIntegerOverflow=on  SampleTime=Ts  OutDataTypeStr=Inherit: Same as first input
  Sum6 : Sum  InputSameDT=on  SaturateOnIntegerOverflow=on  SampleTime=Ts  OutDataTypeStr=Inherit: Same as first input
  Switch : Switch  Criteria=u2 > Threshold  SaturateOnIntegerOverflow=off  InputSameDT=off
  Zero-Order Hold : ZeroOrderHold  SampleTime=Ts
  Out : Outport  SampleTime=Ts  InitialOutput=0  VectorParamsAs1DForOutWhenUnconnected=off
  wires:
  Kp5/1 -> Switch/3
  Switch/1 -> Discrete-Time Integrator/1
  Saturation2/1 -> Out/1
  Discrete-Time Integrator/1 -> Sum6/2
  Kp4/1 -> Zero-Order Hold/1
  Sum6/1 -> Saturation2/1
  Error/1 -> Kp5/1, Kp4/1, Compare To Zero/1, Compare To Zero1/1
  Compare To Zero1/1 -> Logical Operator1/2  "Error_is_negative"
  Logical Operator1/1 -> Logical Operator2/2
  Logical Operator/1 -> Logical Operator2/1
  Compare To Zero/1 -> Logical Operator/2  "Error_is_positive"
  Constant3/1 -> Relational Operator1/2
  Constant1/1 -> Relational Operator/2
  Relational Operator1/1 -> Logical Operator1/1  "LowerLimit_Is_Reached"
  Relational Operator/1 -> Logical Operator/1  "UpperLimit_is_Reached"
  Logical Operator2/1 -> Switch/2
  Sum1/1 -> Relational Operator/1, Relational Operator1/1
  Discrete-Time Integrator/State -> Sum1/1
  Zero-Order Hold/1 -> Sum6/1, Sum1/2
  Constant/1 -> Switch/1

== system B2B_HVDC_MMC/Dq0 Control8/Subsystem/Outer loop - AC RMS controller1/PI regulator with anti-windup Q1 ==
  note: Anti-windup mechanism: Method of conditionnal integration
      |
      | The integration is suspended if saturation occurs and the
      | control error is of the same sign as the control signal.
      |
      | [1] L.Rundqwist, "Anti-Reset Windup for PID Controllers," Ph.D. Thesis TRFT-1033,
      | Departement of Automatic Control, Lund Institute of Technology, Lund, Sweeden, 1991.
  Error : Inport  SampleTime=Ts
  Compare To Zero : simulink/Logic and Bit Operations/Compare To Zero  relop=>  OutDataTypeStr=uint8  ZeroCross=off
  Compare To Zero1 : simulink/Logic and Bit Operations/Compare To Zero  relop=<  OutDataTypeStr=uint8  ZeroCross=off
  Constant : Constant  Value=0
  Constant2 : Constant  Value=UpperLimit
  Constant3 : Constant  Value=LowerLimit
  Discrete-Time Integrator1 : DiscreteIntegrator  IntegratorMethod=Integration: Trapezoidal  InitialCondition=Init  SampleTime=Ts  LimitOutput=on  UpperSaturationLimit=UpperLimit  LowerSaturationLimit=LowerLimit  ShowStatePort=on  ICPrevOutput=DiscIntNeverNeededParam  ICPrevScaledInput=DiscIntNeverNeededParam
  Kp4 : Gain  Gain=Kp  SaturateOnIntegerOverflow=on  SampleTime=Ts  OutDataTypeStr=Inherit: Same as input  ParamDataTypeStr=Inherit: Same as input
  Kp5 : Gain  Gain=Ki  SaturateOnIntegerOverflow=on  SampleTime=Ts  OutDataTypeStr=Inherit: Same as input  ParamDataTypeStr=Inherit: Same as input
  Logical Operator : Logic  AllPortsSameDT=off  OutDataTypeStr=boolean
  Logical Operator1 : Logic  AllPortsSameDT=off  OutDataTypeStr=boolean
  Logical Operator2 : Logic  Operator=OR  AllPortsSameDT=off  OutDataTypeStr=boolean
  Relational Operator : RelationalOperator  OutDataTypeStr=boolean  InputSameDT=off
  Relational Operator1 : RelationalOperator  Operator=<=  OutDataTypeStr=boolean  InputSameDT=off
  Sum1 : Sum  InputSameDT=on  SaturateOnIntegerOverflow=on  SampleTime=Ts  OutDataTypeStr=Inherit: Same as first input
  Sum6 : Sum  InputSameDT=on  SaturateOnIntegerOverflow=on  SampleTime=Ts  OutDataTypeStr=Inherit: Same as first input
  Switch : Switch  Criteria=u2 > Threshold  SaturateOnIntegerOverflow=off  InputSameDT=off
  Zero-Order Hold : ZeroOrderHold  SampleTime=Ts
  Out : Outport  SampleTime=Ts  InitialOutput=0  VectorParamsAs1DForOutWhenUnconnected=off
  wires:
  Constant3/1 -> Relational Operator1/2
  Constant2/1 -> Relational Operator/2
  Sum6/1 -> Out/1
  Discrete-Time Integrator1/State -> Sum1/1
  Discrete-Time Integrator1/1 -> Sum6/2
  Constant/1 -> Switch/1
  Zero-Order Hold/1 -> Sum1/2, Sum6/1
  Sum1/1 -> Relational Operator1/1, Relational Operator/1
  Logical Operator2/1 -> Switch/2
  Relational Operator/1 -> Logical Operator/1  "UpperLimit_is_Reached"
  Relational Operator1/1 -> Logical Operator1/1  "LowerLimit_Is_Reached"
  Compare To Zero/1 -> Logical Operator/2  "Error_is_positive"
  Logical Operator/1 -> Logical Operator2/1
  Logical Operator1/1 -> Logical Operator2/2
  Compare To Zero1/1 -> Logical Operator1/2  "Error_is_negative"
  Error/1 -> Compare To Zero1/1, Compare To Zero/1, Kp4/1, Kp5/1
  Kp4/1 -> Zero-Order Hold/1
  Switch/1 -> Discrete-Time Integrator1/1
  Kp5/1 -> Switch/3

== matlab function B2B_HVDC_MMC/MMC Converter8/MATLAB Function1 ==
  data: x input; z output; y input; dt parameter
function z  = fcn(x,y, dt)

    z = zeros(3,1);
    e = zeros(3,1);


    persistent dt2;
    persistent eo;
    persistent xo;
    persistent yo;
    persistent zo;
    
    
    if(isempty(dt2))
        dt2     = dt/2; 
        xo = zeros(3,1);
        yo = zeros(3,1);
        eo = zeros(3,1);
    end
    

    z = dt*(xo.*yo.^2)+eo.*yo;
    xo = x;
    yo = y;
    eo = eo + dt*(xo.*yo);
    
    %z = e.*y;
    
end

== matlab function B2B_HVDC_MMC/MMC Converter8/MATLAB Function2 ==
  data: x input; z output; y input; dt parameter
function z  = fcn(x,y, dt)

    z = zeros(3,1);
    e = zeros(3,1);


    persistent dt2;
    persistent eo;
    persistent xo;
    persistent yo;
    persistent zo;
    
    
    if(isempty(dt2))
        dt2     = dt/2; 
        xo = zeros(3,1);
        yo = zeros(3,1);
        eo = zeros(3,1);
    end
    

    z = dt*(xo.*yo.^2)+eo.*yo;
    xo = x;
    yo = y;
    eo = eo + dt*(xo.*yo);
    
    %z = e.*y;
    
end

== matlab function B2B_HVDC_MMC/MMC Converter8/MATLAB Function3 ==
  data: x input; z output; y input; dt parameter
function z  = fcn(x,y, dt)

    z = zeros(3,1);
    e = zeros(3,1);


    persistent dt2;
    persistent eo;
    persistent xo;
    persistent yo;
    persistent zo;
    
    
    if(isempty(dt2))
        dt2     = dt/2; 
        xo = zeros(3,1);
        yo = zeros(3,1);
        eo = zeros(3,1);
    end
    

    z = dt*(xo.*yo.^2)+eo.*yo;
    xo = x;
    yo = y;
    eo = eo + dt*(xo.*yo);
    
    %z = e.*y;
    
end

== matlab function B2B_HVDC_MMC/MMC Converter8/MATLAB Function4 ==
  data: x input; z output; y input; dt parameter
function z  = fcn(x,y, dt)

    z = zeros(3,1);
    e = zeros(3,1);


    persistent dt2;
    persistent eo;
    persistent xo;
    persistent yo;
    persistent zo;
    
    
    if(isempty(dt2))
        dt2     = dt/2; 
        xo = zeros(3,1);
        yo = zeros(3,1);
        eo = zeros(3,1);
    end
    

    z = dt*(xo.*yo.^2)+eo.*yo;
    xo = x;
    yo = y;
    eo = eo + dt*(xo.*yo);
    
    %z = e.*y;
    
end

== matlab function B2B_HVDC_MMC/MMC Converter4/MATLAB Function2 ==
  data: Ydcpnz_c output; X_DQN input
function Ydcpnz_c  = fDQN012C(X_DQN)
        
            if(size(X_DQN,2) < 1)
                error('Wrong size!');
            end
            
            N = size(X_DQN,1);
        
            if(size(X_DQN,1) == 6 && size(X_DQN,2) == 1)
                N = 1;
                X_DQN = X_DQN';
            end
        
            Ydcpnz_c = complex(zeros(3,N));
        
            for i = 1 : N
             
                if(i>1)
                    Ydcpnz_c(1,i) = (X_DQN(i,1)) + 1i*X_DQN(i,4);
                    Ydcpnz_c(2,i) = (-X_DQN(i,2)) + 1i*X_DQN(i,5);
                    Ydcpnz_c(3,i) = (X_DQN(i,3)) + 1i*X_DQN(i,6);
                else
        
                    Ydcpnz_c(1,i) = 0.5*(X_DQN(i,4) - 1i*X_DQN(i,1));
                    Ydcpnz_c(2,i) = 0.5*(X_DQN(i,5) + 1i*X_DQN(i,2));
                    Ydcpnz_c(3,i) =     (X_DQN(i,6) + 1i*X_DQN(i,3));
                end
            
            end
        
        
end

== matlab function B2B_HVDC_MMC/MMC Converter4/MATLAB Function3 ==
  data: Ydcpnz_c output; X_DQN input
function Ydcpnz_c  = fDQN012C(X_DQN)
        
            if(size(X_DQN,2) < 1)
                error('Wrong size!');
            end
            
            N = size(X_DQN,1);
        
            if(size(X_DQN,1) == 6 && size(X_DQN,2) == 1)
                N = 1;
                X_DQN = X_DQN';
            end
        
            Ydcpnz_c = complex(zeros(3,N));
        
            for i = 1 : N
             
                if(i>1)
                    Ydcpnz_c(1,i) = (X_DQN(i,1)) + 1i*X_DQN(i,4);
                    Ydcpnz_c(2,i) = (-X_DQN(i,2)) + 1i*X_DQN(i,5);
                    Ydcpnz_c(3,i) = (X_DQN(i,3)) + 1i*X_DQN(i,6);
                else
        
                    Ydcpnz_c(1,i) = 0.5*(X_DQN(i,4) - 1i*X_DQN(i,1));
                    Ydcpnz_c(2,i) = 0.5*(X_DQN(i,5) + 1i*X_DQN(i,2));
                    Ydcpnz_c(3,i) =     (X_DQN(i,6) + 1i*X_DQN(i,3));
                end
            
            end
        
        
end

== matlab function B2B_HVDC_MMC/MMC Converter4/MATLAB Function4 ==
  data: Ydcpnz_c output; X_DQN input
function Ydcpnz_c  = fDQN012C(X_DQN)
        
            if(size(X_DQN,2) < 1)
                error('Wrong size!');
            end
            
            N = size(X_DQN,1);
        
            if(size(X_DQN,1) == 6 && size(X_DQN,2) == 1)
                N = 1;
                X_DQN = X_DQN';
            end
        
            Ydcpnz_c = complex(zeros(3,N));
        
            for i = 1 : N
             
                if(i>1)
                    Ydcpnz_c(1,i) = (X_DQN(i,1)) + 1i*X_DQN(i,4);
                    Ydcpnz_c(2,i) = (-X_DQN(i,2)) + 1i*X_DQN(i,5);
                    Ydcpnz_c(3,i) = (X_DQN(i,3)) + 1i*X_DQN(i,6);
                else
        
                    Ydcpnz_c(1,i) = 0.5*(X_DQN(i,4) - 1i*X_DQN(i,1));
                    Ydcpnz_c(2,i) = 0.5*(X_DQN(i,5) + 1i*X_DQN(i,2));
                    Ydcpnz_c(3,i) =     (X_DQN(i,6) + 1i*X_DQN(i,3));
                end
            
            end
        
        
end

== matlab function B2B_HVDC_MMC/MMC Converter4/MATLAB Function5 ==
  data: Ydcpnz_c output; X_DQN input
function Ydcpnz_c  = fDQN012C(X_DQN)
        
            if(size(X_DQN,2) < 1)
                error('Wrong size!');
            end
            
            N = size(X_DQN,1);
        
            if(size(X_DQN,1) == 6 && size(X_DQN,2) == 1)
                N = 1;
                X_DQN = X_DQN';
            end
        
            Ydcpnz_c = complex(zeros(3,N));
        
            for i = 1 : N
             
                if(i>1)
                    Ydcpnz_c(1,i) = (X_DQN(i,1)) + 1i*X_DQN(i,4);
                    Ydcpnz_c(2,i) = (-X_DQN(i,2)) + 1i*X_DQN(i,5);
                    Ydcpnz_c(3,i) = (X_DQN(i,3)) + 1i*X_DQN(i,6);
                else
        
                    Ydcpnz_c(1,i) = 0.5*(X_DQN(i,4) - 1i*X_DQN(i,1));
                    Ydcpnz_c(2,i) = 0.5*(X_DQN(i,5) + 1i*X_DQN(i,2));
                    Ydcpnz_c(3,i) =     (X_DQN(i,6) + 1i*X_DQN(i,3));
                end
            
            end
        
        
end

== matlab function B2B_HVDC_MMC/MMC Converter4/MATLAB Function6 ==
  data: Ydcpnz_c output; X_DQN input
function Ydcpnz_c  = fDQN012C(X_DQN)
        
            if(size(X_DQN,2) < 1)
                error('Wrong size!');
            end
            
            N = size(X_DQN,1);
        
            if(size(X_DQN,1) == 6 && size(X_DQN,2) == 1)
                N = 1;
                X_DQN = X_DQN';
            end
        
            Ydcpnz_c = complex(zeros(3,N));
        
            for i = 1 : N
             
                if(i>1)
                    Ydcpnz_c(1,i) = (X_DQN(i,1)) + 1i*X_DQN(i,4);
                    Ydcpnz_c(2,i) = (-X_DQN(i,2)) + 1i*X_DQN(i,5);
                    Ydcpnz_c(3,i) = (X_DQN(i,3)) + 1i*X_DQN(i,6);
                else
        
                    Ydcpnz_c(1,i) = 0.5*(X_DQN(i,4) - 1i*X_DQN(i,1));
                    Ydcpnz_c(2,i) = 0.5*(X_DQN(i,5) + 1i*X_DQN(i,2));
                    Ydcpnz_c(3,i) =     (X_DQN(i,6) + 1i*X_DQN(i,3));
                end
            
            end
        
        
end

== matlab function B2B_HVDC_MMC/MMC Converter4/MATLAB Function7 ==
  data: Ydcpnz_c output; X_DQN input
function Ydcpnz_c  = fDQN012C(X_DQN)
        
            if(size(X_DQN,2) < 1)
                error('Wrong size!');
            end
            
            N = size(X_DQN,1);
        
            if(size(X_DQN,1) == 6 && size(X_DQN,2) == 1)
                N = 1;
                X_DQN = X_DQN';
            end
        
            Ydcpnz_c = complex(zeros(3,N));
        
            for i = 1 : N
             
                if(i>1)
                    Ydcpnz_c(1,i) = (X_DQN(i,1)) + 1i*X_DQN(i,4);
                    Ydcpnz_c(2,i) = (-X_DQN(i,2)) + 1i*X_DQN(i,5);
                    Ydcpnz_c(3,i) = (X_DQN(i,3)) + 1i*X_DQN(i,6);
                else
        
                    Ydcpnz_c(1,i) = 0.5*(X_DQN(i,4) - 1i*X_DQN(i,1));
                    Ydcpnz_c(2,i) = 0.5*(X_DQN(i,5) + 1i*X_DQN(i,2));
                    Ydcpnz_c(3,i) =     (X_DQN(i,6) + 1i*X_DQN(i,3));
                end
            
            end
        
        
end
